simulink model "solarmod1507"  (R2018a)
settings: Solver=VariableStepAuto  StartTime=0.0  StopTime=10.0  RelTol=1e-3
undefined symbols (not defined in the file or in its folder): sigbuilder_block
libraries: powerlib x9, re_lib x1, powerlib_meascontrol x1
settings Model: Creator=CC  LastModifiedBy=CC

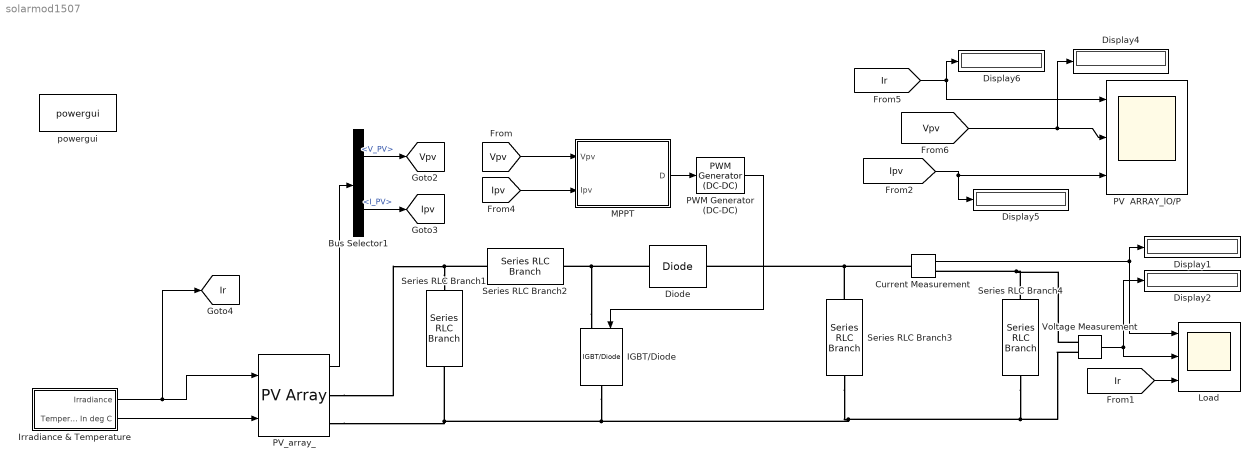
== system solarmod1507 ==
  Bus Selector1 : BusSelector  OutputSignals=V_PV,I_PV
  Current Measurement : powerlib/Measurements/Current Measurement  PhasorSimulation=off  OutputType=Complex  PSBequivalent=0
  Diode : powerlib/Power Electronics/Diode  Ron=0.001  Lon=0  Vf=0.8  IC=0  UseSnubber=0  Rs=500  Cs=250e-9  Measurements=off
  Display{1..2,4..6} (5 alike) : Display
  IGBT/Diode : powerlib/Power Electronics/IGBT//Diode  Ron=1e-3  Rs=1e5  Cs=inf  Measurements=off
  Irradiance & Temperature : Subsystem  Tag=STV Subsys  LoadFcn=sigbuilder_block('load',[437.4 186 550.8 400.2 ]);  StartFcn=sigbuilder_block('start');  StopFcn=sigbuilder_block('stop');  ClipboardFcn=sigbuilder_block('clipboard');  mask(Sigbuilder block){tuvar=[0:10]}
      mask help: Simulink:masks:SigbuilderBlock_MD
      mask init:
      | if ~strcmp(get_param(bdroot(gcbh),'SimulationStatus'),'stopped') tuvar = sigbuilder_block('maskInit'); end
      settings: CopyFcn=sigbuilder_block('copy');  DeleteFcn=sigbuilder_block('delete');  ModelCloseFcn=sigbuilder_block('modelClose');  PreSaveFcn=sigbuilder_block('preSave');  PauseFcn=sigbuilder_block('pause');  ContinueFcn=sigbuilder_block('continue');  NameChangeFcn=sigbuilder_block('namechange');  OpenFcn=sigbuilder_block('open',[437.4 186 550.8 400.2 ]);  CloseFcn=sigbuilder_block('close');
      mask Display: plot(0, 0, 100, 100,[2, 2, 32, 32, 2], [68, 8, 8, 68, 68],[32, 2], [38, 38], [32, 19, 2],[53, 60, 44], [32, 17, 17, 2],[16, 16, 31, 31]);txt = getActiveGroup(gcbh);text(2, 100, txt,'verticalAlignment', 'top');
  Load : Scope  NumInputPorts=3
  MPPT : MATLAB Function  TreatAsAtomicUnit=on
  PV  ARRAY_lO/P : Scope  NumInputPorts=3
  PV_array_ : re_lib/Solar/PV Array  Npar=2  Nser=5  PlotType=array @ 1000 W/m2 & specified temperatures  S_vec="[ 1000  500  100 ]"  Temp_C_vec="[ 45 25  ]"  ModuleName=User-defined  PlotWhenSelected=off  Pm=200.112  Ncell=60  Voc=32.9  Isc=8.21  Vm=26.4  Im=7.58  beta_Voc_pc=-0.35339  alpha_Isc_pc=0.055349  beta_Voc=-0.11627  alpha_Isc=0.0045442  IL=8.232  I0=2.1756e-10  nI=0.87743  Rsh=123.7196  Rs=0.3317  BAL=on  Tc=1e-6  Tfilter=5e-5
  PWM Generator (DC-DC) : powerlib_meascontrol/Pulse & Signal Generators/PWM Generator (DC-DC)  Fsw=5000  Ts=10e-6
  Series RLC Branch1 : powerlib/Elements/Series RLC Branch  LConnTagsString=__new0  RConnTagsString=__new0  BranchType=RC  Resistance=1e-4  Inductance=1e-3  SetiL0=off  InitialCurrent=0  Capacitance=100e-6  Setx0=off  InitialVoltage=0  Measurements=None
  Series RLC Branch2 : powerlib/Elements/Series RLC Branch  LConnTagsString=__new0  RConnTagsString=__new0  BranchType=RL  Resistance=0.1  Inductance=5e-3  SetiL0=off  InitialCurrent=0  Capacitance=100e-6  Setx0=off  InitialVoltage=0  Measurements=None
  Series RLC Branch3 : powerlib/Elements/Series RLC Branch  LConnTagsString=__new0  RConnTagsString=__new0  BranchType=RC  Resistance=1e-4  Inductance=1e-3  SetiL0=off  InitialCurrent=0  Capacitance=3300e-6  Setx0=off  InitialVoltage=0  Measurements=None
  Series RLC Branch4 : powerlib/Elements/Series RLC Branch  LConnTagsString=__new0  RConnTagsString=__new0  BranchType=R  Resistance=8.6  Inductance=1e-3  SetiL0=off  InitialCurrent=0  Capacitance=3300e-6  Setx0=off  InitialVoltage=0  Measurements=None
  Voltage Measurement : powerlib/Measurements/Voltage Measurement  PhasorSimulation=off  OutputType=Complex  PSBequivalent=0
  powergui : powerlib/powergui  Priority=1  SimulationMode=Discrete  SampleTime=1e-6  frequency=60  Iterations=50  frequencyindice=0  Pbase=100e6  ErrMax=1e-4  UnitsV=kV  UnitsW=MW  buscounter=0  FunctionMessages=off  echomessages=off  EnableUseOfTLC=off  CurrentSourceSwitches=off  DisableSnubberDevices=off  DisableRonSwitches=off  DisableVfSwitches=off  DisplayEquations=off  SolverType=Tustin/Backward Euler (TBE)  Interpol=off  ExternalGateDelay=off  methode=off  Ts=100  x0status=blocks  SPID=on  SwTol=0  HookPort=off  RestoreLinks=warning  ResistiveCurrentMeasurement=off  Frange=[0:2:500]  Ylog=off  Xlog=on  ShowGrid=off  save=off  variable=ZData  structure=0  ZoomFFT=off  StartTime=0.0  cycles=1  DisplayStyle=1  fundamental=60  FreqAxis=off  MaxFrequency=1000  frequencyindicesteady=1  RmsSteady=1  display=off
  tag scope: Ipv=global, Ir=global, Vpv=global
  wires:
  [Ipv] -> MPPT/2(Ipv)
  MPPT/1(D) -> PWM Generator (DC-DC)/1
  [Vpv] -> MPPT/1(Vpv)
  PWM Generator (DC-DC)/1 -> IGBT/Diode/1
  [Ipv] -> Display5/1, PV  ARRAY_lO/P/3
  [Vpv] -> Display4/1, PV  ARRAY_lO/P/2
  PV_array_/1 -> Bus Selector1/1
  Bus Selector1/2 -> [Ipv]  "<I_PV>"
  Bus Selector1/1 -> [Vpv]  "<V_PV>"
  [Ir] -> PV  ARRAY_lO/P/1, Display6/1
  Current Measurement/1 -> Display1/1, Load/1
  Voltage Measurement/1 -> Load/2, Display2/1
  [Ir] -> Load/3
  Irradiance & Temperature/1(Irradiance) -> [Ir], PV_array_/1
  Irradiance & Temperature/2(Temperature In deg C) -> PV_array_/2
  connections:
  IGBT/Diode/LConn1 -- Diode/LConn1 -- Series RLC Branch2/RConn1
  PV_array_/RConn2 -- Series RLC Branch4/RConn1 -- Voltage Measurement/LConn2 -- Series RLC Branch3/RConn1 -- IGBT/Diode/RConn1 -- Series RLC Branch1/RConn1
  Series RLC Branch1/LConn1 -- PV_array_/RConn1 -- Series RLC Branch2/LConn1
  Series RLC Branch3/LConn1 -- Current Measurement/LConn1 -- Diode/RConn1
  Series RLC Branch4/LConn1 -- Voltage Measurement/LConn1 -- Current Measurement/RConn1

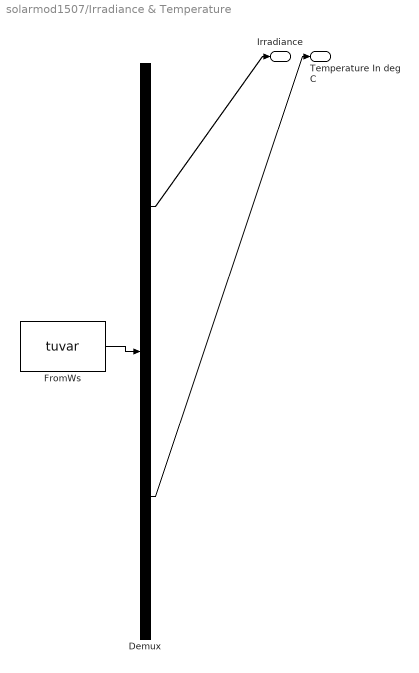
== system solarmod1507/Irradiance & Temperature ==
  Demux : Demux  Tag=STV Demux  Outputs=2
  FromWs : FromWorkspace  Tag=STV FromWs  VariableName=tuvar  SampleTime=0
      SigBuilderData=|
      | common.afterFinalStr = 'Extrapolate'
      | common.sampleTime = 0
      | dataSet.timeRange = [0 10]
      | dataSet.name = 'Group 1'
      | sbobj.Groups.Name = 'Group 1'
      | sbobj.Groups.Signals(1).Name = 'Irradiance'
      | sbobj.Groups.Signals(1).XData = [0 1 2 3 4 5 6 7 8 9 10]
      | sbobj.Groups.Signals(1).YData = [479.77 479.77 677.52 830.62 932.02 945.27 904.4 798.17 635.35 435.02 228.08]
      | sbobj.Groups.Signals(2).Name = 'Temperature In deg C'
      | sbobj.Groups.Signals(2).XData = [0 1 2 3 4 5 6 7 8 9 10]
      | sbobj.Groups.Signals(2).YData = [33.41 33.41 36.94 39.58 41.26 42.55 43.5 43.98 43.88 43.29 42.17]
  Irradiance : Outport  Tag=STV Outport
  Temperature In deg C : Outport  Tag=STV Outport  Port=2
  wires:
  FromWs/1 -> Demux/1
  Demux/1 -> Irradiance/1
  Demux/2 -> Temperature In deg C/1

== matlab function solarmod1507/MPPT ==
  data: Vpv input; D output; Ipv input
function D = Pand0(Vpv,Ipv)



persistent Dprev Pprev Vprev

if isempty (Dprev) 
   
Dprev = 0.7;

Vprev = 190;

Pprev = 2000;

end

deltaD = 125e-6;

% Calculate measured array power

Ppv = Vpv*Ipv;

% Increase or decrease duty cycle based on conditions

if (Ppv-Pprev) ~= 0 
    if (Ppv-Pprev) > 0

if (Vpv-Vprev) > 0

D= Dprev - deltaD;

else

D = Dprev + deltaD;

end

else

if (Vpv-Vprev) > 0

D= Dprev + deltaD;

else

D = Dprev - deltaD;

end
    end
else
    D = Dprev;
end
% Update internal values

Dprev = D;

Vprev = Vpv; 

Pprev = Ppv;
